simulink model "ex8"  (Simulink 6.0)
settings: Solver=ode45  StartTime=0.0  StopTime=5  MaxStep=0.001  RelTol=1e-3
undefined symbols (not defined in the file or in its folder): magnitude
libraries: commanapbnd2 x3, dsparch4 x2, commchan2 x1, dspstat3 x1, commrandsrc2 x1
settings Model: LastModifiedBy=lxy

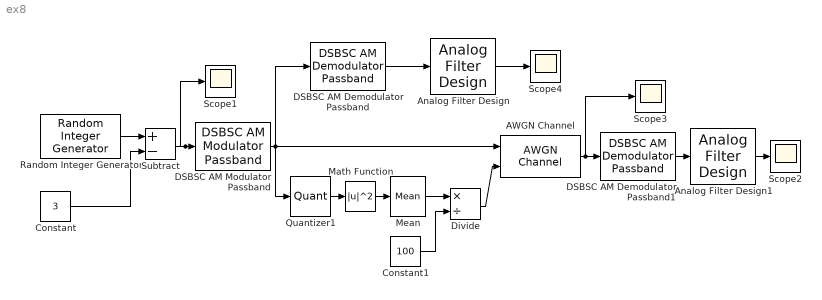
== system ex8 ==
  AWGN Channel : commchan2/AWGN Channel  seed=67  noiseMode=Variance from port  EbNodB=10  EsNodB=10  SNRdB=10  bitsPerSym=1  Ps=1  Tsym=1  variance=1
  Analog Filter Design : dsparch4/Analog Filter Design  method=Bessel  filttype=Lowpass  N=8  Wlo=2*pi*100  Whi=80  Rp=1  Rs=40
  Analog Filter Design1 : dsparch4/Analog Filter Design  method=Bessel  filttype=Lowpass  N=8  Wlo=2*pi*100  Whi=80  Rp=2  Rs=40
  Constant : Constant  Value=3
  Constant1 : Constant  Value=100
  DSBSC AM Demodulator Passband : commanapbnd2/DSBSC AM Demodulator Passband  Fc=100  num=[4.57 9.14 4.57]*.01  den=[1 -1.3108 .4936]  Ph=pi/2  ts=0.001
  DSBSC AM Demodulator Passband1 : commanapbnd2/DSBSC AM Demodulator Passband  Fc=100  num=[4.57 9.14 4.57]*.01  den=[1 -1.3108 .4936]  Ph=pi/2  ts=0.001
  DSBSC AM Modulator Passband : commanapbnd2/DSBSC AM Modulator Passband  Fc=100  Ph=pi/2
  Divide : Product  Inputs=*/  OutScaling=2^-10
  Math Function : Math  Operator=magnitude^2  SaturateOnIntegerOverflow=on
  Mean : dspstat3/Mean  DialogController=dspDDGCreate  DialogControllerArgs=DataTag0  run=on  reset_popup=None  roundingMode=Floor  overflowMode=off
  Quantizer1 : Quantizer  QuantizationInterval=0.001  LinearizeAsGain=off  SampleTime=0.001
  Random Integer Generator : commrandsrc2/Random Integer Generator  mul=7  seed=1234  Ts=1/2  frameBased=off  sampPerFrame=1  orient=off
  Scope{1..4} (4 alike) : Scope
      Scope3 settings: YMin=-10  YMax=10  SaveName=ScopeData2
      Scope4 settings: SaveName=ScopeData3
  Subtract : Sum  Inputs=+-  OutScaling=2^-10
  wires:
  Random Integer Generator/1 -> Subtract/1
  Constant/1 -> Subtract/2
  Subtract/1 -> Scope1/1, DSBSC AM Modulator Passband/1
  DSBSC AM Demodulator Passband1/1 -> Analog Filter Design1/1
  DSBSC AM Modulator Passband/1 -> Quantizer1/1, AWGN Channel/1, DSBSC AM Demodulator Passband/1
  Constant1/1 -> Divide/2
  Divide/1 -> AWGN Channel/2
  AWGN Channel/1 -> Scope3/1, DSBSC AM Demodulator Passband1/1
  DSBSC AM Demodulator Passband/1 -> Analog Filter Design/1
  Analog Filter Design/1 -> Scope4/1
  Analog Filter Design1/1 -> Scope2/1
  Math Function/1 -> Mean/1
  Quantizer1/1 -> Math Function/1
  Mean/1 -> Divide/1
